simulink model "dcdc1"  (Simulink 7.5)
settings: Solver=ode23tb  StartTime=0.0  StopTime=0.1  FixedStep=1e-8  RelTol=1e-3
libraries: powerlib x19, simulink x1
settings Model: Creator=kmathew  LastModifiedBy=RISHI

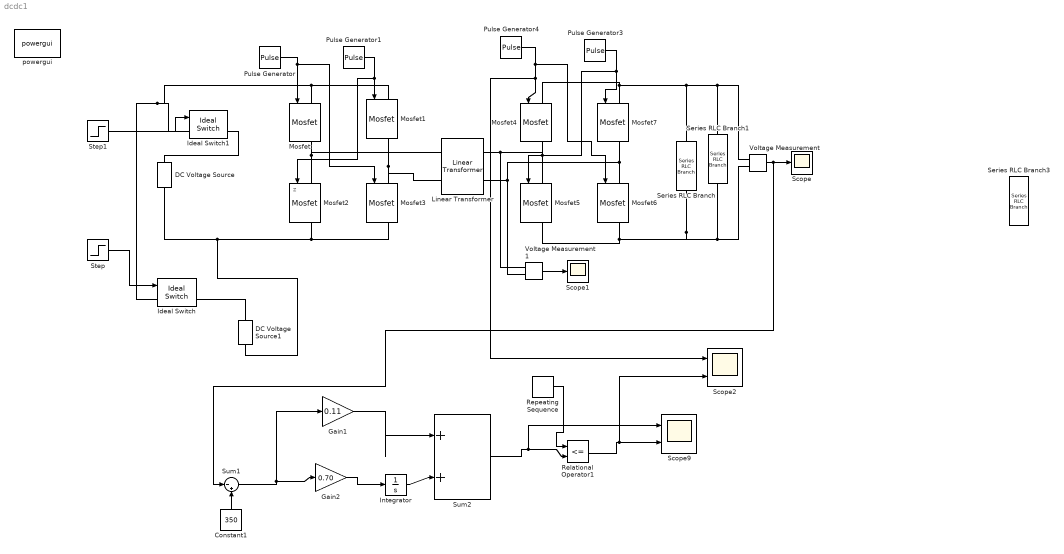
== system dcdc1 ==
  note: z
  Constant1 : Constant  Value=350  OutDataType=fixdt(1, 16)  OutScaling=2^0
  DC Voltage Source : powerlib/Electrical Sources/DC Voltage Source  DialogController=POWERSYS.PowerSysDialog  SystemSampleTime=-1  Amplitude=72  Measurements=None
  DC Voltage Source1 : powerlib/Electrical Sources/DC Voltage Source  DialogController=POWERSYS.PowerSysDialog  SystemSampleTime=-1  Amplitude=3  Measurements=None
  Gain1 : Gain  Gain=0.11  ParameterDataType=sfix(16)  ParameterScaling=2^0  OutDataType=sfix(16)  OutScaling=2^0
  Gain2 : Gain  Gain=0.70  ParameterDataType=sfix(16)  ParameterScaling=2^0  OutDataType=sfix(16)  OutScaling=2^0
  Ideal Switch : powerlib/Power Electronics/Ideal Switch  DialogController=POWERSYS.PowerSysDialog  SystemSampleTime=-1  Ron=0.001  Lon=0  IC=0  Rs=1e5  Cs=inf  Measurements=on
  Ideal Switch1 : powerlib/Power Electronics/Ideal Switch  DialogController=POWERSYS.PowerSysDialog  SystemSampleTime=-1  Ron=0.001  Lon=0  IC=0  Rs=1e5  Cs=inf  Measurements=on
  Integrator : Integrator
  Linear Transformer : powerlib/Elements/Linear Transformer  DialogController=POWERSYS.PowerSysDialog  PhysicalDomain=powersysdomain  SubClassName=unknown  LeftPortType=p1  RightPortType=p1  LConnTagsString=a|b  RConnTagsString=A|B  UNITS=SI  NominalPower=[8e3 20000 ]  winding1=[100 0.00025 0]  winding2=[486 0.0004 0]  ThreeWindings=off  winding3=[3.15e+05 24806 7.8961]  RmLm=[1000 360e-6]  Measurements=None  DataType=on
  Mosfet{,1..3} (4 alike) : powerlib/Power Electronics/Mosfet  DialogController=POWERSYS.PowerSysDialog  SystemSampleTime=-1  Ron=2e-3  Lon=0  Rd=2e-3  Vfd=1  IC=0  Rs=1e5  Cs=inf  Measurements=on
  Mosfet{4..7} (4 alike) : powerlib/Power Electronics/Mosfet  DialogController=POWERSYS.PowerSysDialog  SystemSampleTime=-1  Ron=5e-3  Lon=0  Rd=5e-3  Vfd=1  IC=0  Rs=1e5  Cs=inf  Measurements=on
  Pulse Generator : DiscretePulseGenerator  PulseType=Time based  Amplitude=5  Period=50e-6  PulseWidth=50  PhaseDelay=0  SampleTime=1
  Pulse Generator1 : DiscretePulseGenerator  PulseType=Time based  Amplitude=5  Period=50e-6  PulseWidth=50  PhaseDelay=25e-6  SampleTime=1
  Pulse Generator3 : DiscretePulseGenerator  PulseType=Time based  Amplitude=5  Period=50e-6  PulseWidth=50  PhaseDelay=25e-6  SampleTime=1
  Pulse Generator4 : DiscretePulseGenerator  PulseType=Time based  Amplitude=5  Period=50e-6  PulseWidth=50  PhaseDelay=0  SampleTime=1
  Relational Operator1 : RelationalOperator  Operator=<=  LogicOutDataTypeMode=boolean  LogicDataType=fixdt(0, 8)  OutDataTypeStr=boolean
  Repeating Sequence : simulink/Sources/Repeating Sequence  SystemSampleTime=-1  rep_seq_t=[0 20e-6]  rep_seq_y=[0 15]
  Scope : Scope
      settings: YMin=329.984  YMax=364.72  Decimation=20
  Scope1 : Scope
      settings: YMin=0.153  YMax=0.1595  Decimation=20
  Scope2 : Scope  NumInputPorts=2
      settings: TimeRange=0.05  YMin=1.9~1.89  YMax=2.1~2.05  SaveName=ScopeData3
  Scope9 : Scope  NumInputPorts=2
      settings: TimeRange=0.05  YMin=1.9~1.89  YMax=2.1~2.05  SaveName=ScopeData2
  Series RLC Branch : powerlib/Elements/Series RLC Branch  DialogController=POWERSYS.PowerSysDialog  PhysicalDomain=powersysdomain  SubClassName=unknown  LeftPortType=p1  RightPortType=p1  LConnTagsString=__new0  RConnTagsString=__new0  BranchType=C  Resistance=1  Inductance=1e-3  SetiL0=off  InitialCurrent=0  Capacitance=10000e-6  Setx0=off  InitialVoltage=0  Measurements=Branch voltage
  Series RLC Branch1 : powerlib/Elements/Series RLC Branch  DialogController=POWERSYS.PowerSysDialog  PhysicalDomain=powersysdomain  SubClassName=unknown  LeftPortType=p1  RightPortType=p1  LConnTagsString=__new0  RConnTagsString=__new0  BranchType=R  Resistance=15  Inductance=1e-3  SetiL0=off  InitialCurrent=0  Capacitance=10e-6  Setx0=off  InitialVoltage=0  Measurements=Branch voltage
  Series RLC Branch3 : powerlib/Elements/Series RLC Branch  DialogController=POWERSYS.PowerSysDialog  PhysicalDomain=powersysdomain  SubClassName=unknown  LeftPortType=p1  RightPortType=p1  LConnTagsString=__new0  RConnTagsString=__new0  BranchType=R  Resistance=2e-3  Inductance=1e-3  SetiL0=off  InitialCurrent=0  Capacitance=10e-6  Setx0=off  InitialVoltage=0  Measurements=Branch voltage
  Step : Step  Time=0.05  SampleTime=0
  Step1 : Step  Time=0.05  Before=1  After=0  SampleTime=0
  Sum1 : Sum  Inputs=|-+  OutDataType=sfix(16)  OutScaling=2^0
  Sum2 : Sum  Inputs=|++  OutDataType=sfix(16)  OutScaling=2^0
  Voltage Measurement : powerlib/Measurements/Voltage Measurement  DialogController=POWERSYS.PowerSysDialog  SystemSampleTime=-1  PhasorSimulation=off  OutputType=Complex  PSBequivalent=0
  Voltage Measurement1 : powerlib/Measurements/Voltage Measurement  DialogController=POWERSYS.PowerSysDialog  SystemSampleTime=-1  PhasorSimulation=off  OutputType=Complex  PSBequivalent=0
  powergui : powerlib/powergui  Priority=1  SystemSampleTime=-1  SimulationMode=Continuous  SampleTime=1e-8  frequency=60  SPID=off  DisableSnubberDevices=off  DisableRonSwitches=off  DisableVfSwitches=off  SwTol=0  Interpol=off  frequencyindice=0  echomessages=off  HookPort=off  DisplayEquations=off  FunctionMessages=off  EnableUseOfTLC=off  x0status=blocks  RestoreLinks=warning  ResistiveCurrentMeasurement=off  Ylog=off  Xlog=on  ShowGrid=off  save=off  variable=ZData  ZoomFFT=off  StartTime=0.0  cycles=1  DisplayStyle=1  FreqAxis=off  MaxFrequency=1000  frequencyindicesteady=1  display=off  methode=off
  wires:
  Voltage Measurement/1 -> Scope/1, Sum1/1
  Pulse Generator/1 -> Mosfet/1, Mosfet3/1
  Pulse Generator1/1 -> Mosfet2/1, Mosfet1/1
  Pulse Generator4/1 -> Mosfet4/1, Scope2/1, Mosfet6/1
  Pulse Generator3/1 -> Mosfet5/1, Mosfet7/1
  Voltage Measurement1/1 -> Scope1/1
  Step/1 -> Ideal Switch/1
  Step1/1 -> Ideal Switch1/1
  Gain2/1 -> Integrator/1
  Integrator/1 -> Sum2/2
  Gain1/1 -> Sum2/1
  Sum2/1 -> Relational Operator1/2, Scope9/1
  Repeating Sequence/1 -> Relational Operator1/1
  Relational Operator1/1 -> Scope9/2, Scope2/2
  Sum1/1 -> Gain1/1, Gain2/1
  Constant1/1 -> Sum1/2
  connections:
  Linear Transformer/LConn2 -- Mosfet1/RConn1 -- Mosfet3/LConn1
  Ideal Switch/LConn1 -- Mosfet1/LConn1 -- Mosfet/LConn1 -- Ideal Switch1/LConn1
  Mosfet3/RConn1 -- Mosfet2/RConn1 -- DC Voltage Source/LConn1 -- DC Voltage Source1/LConn1
  Linear Transformer/RConn2 -- Mosfet6/LConn1 -- Mosfet7/RConn1 -- Voltage Measurement1/LConn2
  Linear Transformer/RConn1 -- Mosfet4/RConn1 -- Mosfet5/LConn1 -- Voltage Measurement1/LConn1
  Mosfet6/RConn1 -- Series RLC Branch/RConn1 -- Voltage Measurement/LConn2 -- Series RLC Branch1/RConn1 -- Mosfet5/RConn1
  Voltage Measurement/LConn1 -- Mosfet7/LConn1 -- Mosfet4/LConn1 -- Series RLC Branch/LConn1 -- Series RLC Branch1/LConn1
  Linear Transformer/LConn1 -- Mosfet/RConn1 -- Mosfet2/LConn1
  Ideal Switch/RConn1 -- DC Voltage Source1/RConn1
  Ideal Switch1/RConn1 -- DC Voltage Source/RConn1
